simulink model "Non_Adaptive_Simulation"  (R2018a)
settings: Solver=VariableStepAuto  StartTime=0.0  StopTime=2  RelTol=1e-3
values from neighbouring files (symbols this model uses):
  AT_filt_U = [0 1;-t2 -t1]    [Adaptive_Script.m]    (also in Non_Adaptive_Script.m)
  AT_filt_Y = [0 1;-t2 -t1]    [Adaptive_Script.m]    (also in Non_Adaptive_Script.m)
  BT_filt_U = [0;1]    [Adaptive_Script.m]    (also in Non_Adaptive_Script.m)
  BT_filt_Y = [0;1]    [Adaptive_Script.m]    (also in Non_Adaptive_Script.m)
  CT_filt_U = [1 0; 0 1]    [Adaptive_Script.m]    (also in Non_Adaptive_Script.m = [G1(2) 0; 0 G1(1)])
  CT_filt_Y = [1 0; 0 1]    [Adaptive_Script.m]    (also in Non_Adaptive_Script.m = [F_bar(2) 0; 0 F_bar(1)])
  Kstar_R = Ref_plant_Km/True_plant_Kp    (= -1000)    [Non_Adaptive_Script.m]
  Ref_plant_Km = 1/time_const    (= 5)    [Adaptive_Script.m]    (also in Non_Adaptive_Script.m = 500)
  Ref_plant_Rm = [1 1/time_const]    [Adaptive_Script.m]    (also in Non_Adaptive_Script.m)
  True_plant_Kp = -0.5    [Adaptive_Script.m]    (also in Non_Adaptive_Script.m)
  True_plant_Rp = [1 0.4 4.3]    [Adaptive_Script.m]    (also in Non_Adaptive_Script.m)
  True_plant_Zp = [1 2]    [Adaptive_Script.m]    (also in Non_Adaptive_Script.m)
settings Model: Creator=ageng  LastModifiedBy=ageng

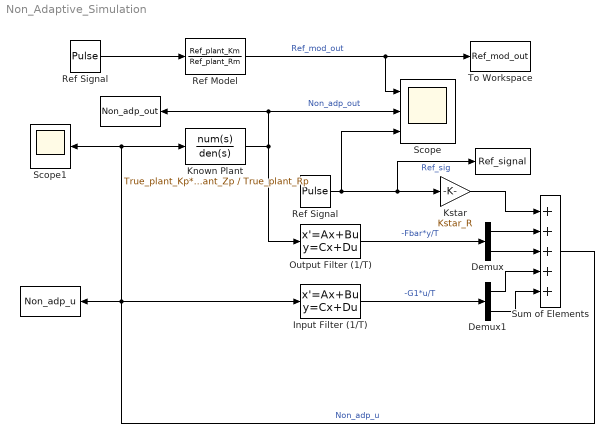
== system Non_Adaptive_Simulation ==
  " " : ToWorkspace  VariableName=Non_adp_out  SaveFormat=Timeseries  SampleTime=0.0001
      settings: Decimation=3
  "  " : ToWorkspace  VariableName=Ref_signal  SaveFormat=Timeseries  SampleTime=0.0001
      settings: Decimation=3
  "     " : ToWorkspace  VariableName=Non_adp_u  SaveFormat=Timeseries  SampleTime=0.0001
      settings: Decimation=3
  Demux : Demux  Outputs=2
  Demux1 : Demux  Outputs=2
  Input Filter (1/T) : StateSpace  A=AT_filt_U  B=BT_filt_U  C=CT_filt_U  D=[0;0]  InitialCondition=0
  Known Plant : TransferFcn  Numerator=True_plant_Kp*True_plant_Zp  Denominator=True_plant_Rp
  Kstar : Gain  Gain=Kstar_R
  Output Filter (1/T) : StateSpace  A=AT_filt_Y  B=BT_filt_Y  C=CT_filt_Y  D=[0;0]  InitialCondition=0
  Ref Model : TransferFcn  Numerator=Ref_plant_Km  Denominator=Ref_plant_Rm
  Ref Signal : DiscretePulseGenerator  PulseType=Time based  Period=1  PulseWidth=50
  "Ref Signal " : DiscretePulseGenerator  PulseType=Time based  Period=1  PulseWidth=50
  Scope : Scope  NumInputPorts=3
  Scope1 : Scope
  Sum of Elements : Sum  Inputs=5
  To Workspace : ToWorkspace  VariableName=Ref_mod_out  SaveFormat=Timeseries  SampleTime=0.0001
      settings: Decimation=3
  wires:
  Known Plant/1 -> " "/1, Scope/2, Output Filter (1/T)/1  "Non_adp_out"
  Output Filter (1/T)/1 -> Demux/1  "-Fbar*y/T"
  Input Filter (1/T)/1 -> Demux1/1  "-G1*u/T"
  Ref Signal/1 -> Scope/3, "  "/1, Kstar/1  "Ref_sig"
  Sum of Elements/1 -> Known Plant/1, Scope1/1, "     "/1, Input Filter (1/T)/1  "Non_adp_u"
  Kstar/1 -> Sum of Elements/1
  Demux/1 -> Sum of Elements/2
  Demux/2 -> Sum of Elements/3
  Demux1/1 -> Sum of Elements/4
  Demux1/2 -> Sum of Elements/5
  "Ref Signal "/1 -> Ref Model/1
  Ref Model/1 -> To Workspace/1, Scope/1  "Ref_mod_out"
